simulink model "q5_simulink"  (R2023b)
settings: Solver=VariableStepAuto  StartTime=0.0  StopTime=15  RelTol=1e-3
values from neighbouring files (symbols this model uses):
  A = [0, 1,      0;       0, -b/J,   K/J;       0, -K/L, -R/L;]    [lec7_dc_motor_control_example.m]    (also in lec7_example_11.m = [0 0 4 1; lec7_notes_example_11.m = [-1, 1, 0;       0,  1, 1;       0,  0, 2;]; mini_proj_1.m = [-8.8487 + (a-b)/5,     -0.0399,              -5.55 + (c+d)/; mini_proj_q1.m = [-8.8487 + (a-b)/5,     -0.0399,              -5.55 + (c+d)/)
  B = [0;       0;       1/L;]    [lec7_dc_motor_control_example.m]    (also in lec7_example_11.m = [-2 0; lec7_notes_example_11.m = [1, 1;       0, 0;       0, 1;]; mini_proj_1.m = [0.0564+(b)/(10+c),           0.0319;       0.0165-(c+d-5)/(; mini_proj_q1.m = [0.0564+(b)/(10+c),           0.0319)
  C = [1, 0, 0]    [lec7_dc_motor_control_example.m]    (also in lec7_notes_example_11.m = [1, 3, -1;      0, 1,  0;]; mini_proj_1.m = [-3.2988,           -2.1932+(10*c+d)/(100+5*a), 0.0370,  -0.; mini_proj_q1.m = [-3.2988,           -2.1932+(10*c+d)/(100+5*a), 0.0370,  -0.; mini_proj_q2.m = [-3.2988,           -2.1932+(10*c+d)/(100+5*a), 0.0370,  -0.)
  C_T_matrix_inv = inv(C_T_matrix)    [q3_full.m]    (also in q5_full.m = [-0.292392890492903   0.278799577693527  -0.115994901359206 )
  D = [0, 0 ... (first row only)    [q1_full.m]    (also in q1_params.m; q2_full.m; q3_full.m = [-1 0; q4_full.m)
  E = T * B    [q3_full.m]    (also in q5_full.m = [-0.179108013653627  -0.106649750104643)
  G = double(subs(G, [struct('g1_1', 1, 'g1_2', 0, 'g2_1', 0, 'g2_2', 1)]))    [q3_full.m]    (also in q5_full.m = [1 0)
  K = transpose(place(A, B, des_poles))    [lec7_dc_motor_control_example.m]    (also in lec7_example_11.m = K_bar * T; lec7_notes_example_11.m = K_bar * T; mini_proj_1.m = K_bar * T; mini_proj_q1.m = K_bar * T)
settings Model: Creator=john  LastModifiedBy=john

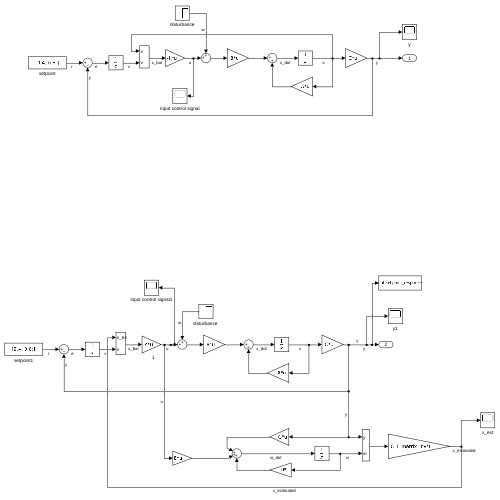
[thumbnail: Simulink's stored preview of the top-level diagram]
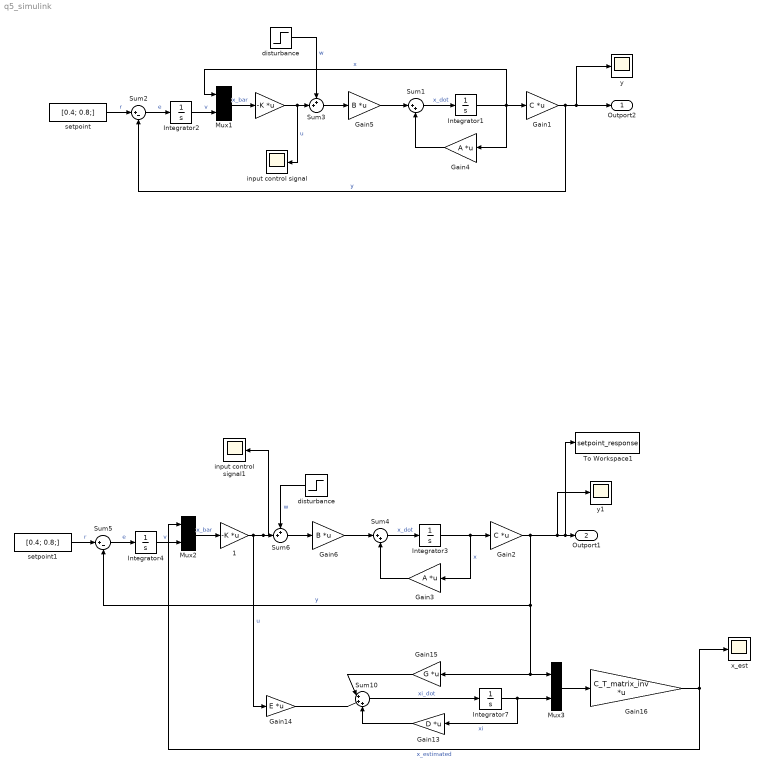
== system q5_simulink ==
  "   " : Gain  Gain=-K  Multiplication=Matrix(K*u)
  "   1" : Gain  Gain=-K  Multiplication=Matrix(K*u)
  Gain1 : Gain  Gain=C  Multiplication=Matrix(K*u)
  Gain13 : Gain  Gain=D  Multiplication=Matrix(K*u)
  Gain14 : Gain  Gain=E  Multiplication=Matrix(K*u)
  Gain15 : Gain  Gain=G  Multiplication=Matrix(K*u)
  Gain16 : Gain  Gain=C_T_matrix_inv  Multiplication=Matrix(K*u)
  Gain2 : Gain  Gain=C  Multiplication=Matrix(K*u)
  Gain3 : Gain  Gain=A  Multiplication=Matrix(K*u)
  Gain4 : Gain  Gain=A  Multiplication=Matrix(K*u)
  Gain5 : Gain  Gain=B  Multiplication=Matrix(K*u)
  Gain6 : Gain  Gain=B  Multiplication=Matrix(K*u)
  Integrator{1..4,7} (5 alike) : Integrator
  Mux1 : Mux  Inputs=2
      settings: DisplayOption=signals
  Mux2 : Mux  Inputs=2
      settings: DisplayOption=signals
  Mux3 : Mux  Inputs=2
      settings: DisplayOption=signals
  Sum1 : Sum  Inputs=|++
  Sum10 : Sum  Inputs=|+++
  Sum2 : Sum  Inputs=|+-
  Sum3 : Sum  Inputs=++|
  Sum4 : Sum  Inputs=|++
  Sum5 : Sum  Inputs=|+-
  Sum6 : Sum  Inputs=++|
  To Workspace1 : ToWorkspace  VariableName=setpoint_response  SaveFormat=Timeseries  SampleTime=-1
  disturbance : Step  Time=10  Before=[0; 0;]  After=[0.3; 0.2;]  SampleTime=0
  "disturbance " : Step  Time=10  Before=[0; 0;]  After=[0.3; 0.2;]  SampleTime=0
  input control signal : Scope
  input control signal1 : Scope
  setpoint : Constant  Value=[0.4; 0.8;]
  setpoint1 : Constant  Value=[0.4; 0.8;]
  x_est : Scope
  y : Scope
  y1 : Scope
  Outport2 : Outport
  Outport1 : Outport  Port=2
  wires:
  disturbance/1 -> Sum3/1  "w"
  Sum3/1 -> Gain5/1
  Gain5/1 -> Sum1/1
  Gain4/1 -> Sum1/2
  Integrator1/1 -> Mux1/1, Gain1/1, Gain4/1  "x"
  Sum2/1 -> Integrator2/1  "e"
  Sum1/1 -> Integrator1/1  "x_dot"
  Gain1/1 -> Sum2/2, y/1, Outport2/1  "y"
  setpoint/1 -> Sum2/1  "r"
  Integrator2/1 -> Mux1/2  "v"
  Mux1/1 -> "   "/1  "x_bar"
  "   "/1 -> input control signal/1, Sum3/2  "u"
  Gain3/1 -> Sum4/2
  Sum5/1 -> Integrator4/1  "e"
  Sum6/1 -> Gain6/1
  Gain6/1 -> Sum4/1
  Sum4/1 -> Integrator3/1  "x_dot"
  setpoint1/1 -> Sum5/1  "r"
  "disturbance "/1 -> Sum6/1  "w"
  Mux2/1 -> "   1"/1  "x_bar"
  Integrator3/1 -> Gain2/1, Gain3/1  "x"
  Integrator4/1 -> Mux2/2  "v"
  Gain13/1 -> Sum10/3
  Sum10/1 -> Integrator7/1  "xi_dot"
  Gain15/1 -> Sum10/1
  Mux3/1 -> Gain16/1
  Gain14/1 -> Sum10/2
  Gain16/1 -> x_est/1, Mux2/1  "x_estimated"
  "   1"/1 -> Gain14/1, input control signal1/1, Sum6/2  "u"
  Integrator7/1 -> Gain13/1, Mux3/2  "xi"
  Gain2/1 -> Mux3/1, Gain15/1, Sum5/2, y1/1, To Workspace1/1, Outport1/1  "y"
